simulink subsystem "VehicleSimulationRef"  (R2024b)
settings: Solver=VariableStepAuto  StartTime=0.0  StopTime=10.0  RelTol=1e-3
undefined symbols (not defined in the file): damp, flightTrajectory, Ka_accel, Kd_rate, Ki_angle, Kp_angle, omega, resetFlag, SimIn, SimPar, trajLen
libraries: starslibAxisTransformations x6, simulink_extras x5, dspstat3 x3, vrlib x3, aerolibanimutils x2, dspnetwork x1, aerolibfltsims x1, simulink x1
(part 1 of 2)
settings Model: Creator=tbritton  LastModifiedBy=edison
settings SolverCC: AlgebraicLoopSolver=TrustRegion
settings OptimizationCC: ReuseModelBlockBuffer=off
settings DebuggingCC: UnconnectedInputMsg=warning  UnconnectedOutputMsg=warning  UnconnectedLineMsg=warning
settings ModelReferenceCC: EnableRefExpFcnMdlSchedulingChecks=on
settings RTWCC: GPUComputeCapability=3.5  DLArmComputeVersion=19.05

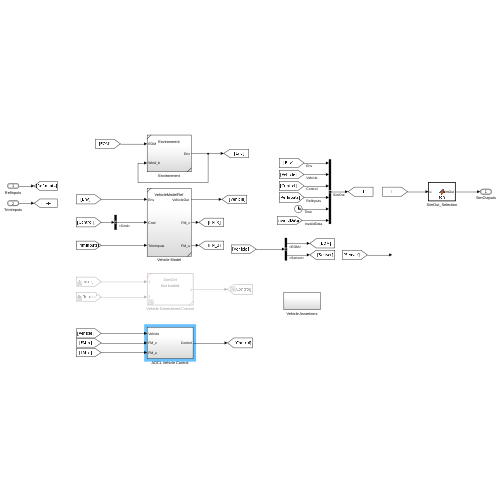
[thumbnail: Simulink's stored preview of the top-level diagram]
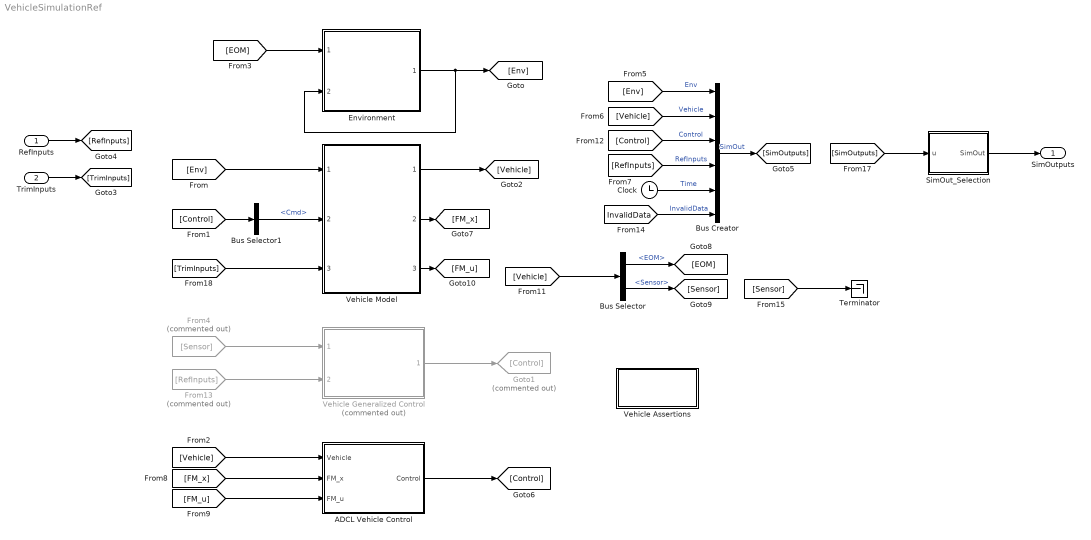
== system VehicleSimulationRef ==
  RefInputs : Inport  OutDataTypeStr=Bus: BUS_REF_INPUT
  TrimInputs : Inport  Port=2  OutDataTypeStr=Bus: BUS_TRIM_INPUT
  ADCL Vehicle Control : Subsystem
  Bus Creator : BusCreator  Inputs=6  OutDataTypeStr=Bus: BUS_SIM_OUT  NonVirtualBus=on
  Bus Selector : BusSelector  OutputSignals=EOM,Sensor
  Bus Selector1 : BusSelector  OutputSignals=Cmd
  Clock : Clock
  Environment : Subsystem  ReferencedSubsystem=Environment
  From13 : From  Commented=on  GotoTag=RefInputs
  From4 : From  Commented=on  GotoTag=Sensor
  Goto1 : Goto  Commented=on  GotoTag=Control
  SimOut_Selection : MATLAB Function  TreatAsAtomicUnit=on
  Terminator : Terminator
  Vehicle Assertions : Subsystem
  Vehicle Generalized Control : Subsystem  Commented=on  ReferencedSubsystem=GenCtrl
  Vehicle Model : Subsystem  ReferencedSubsystem=VehicleModelRef
  SimOutputs : Outport  OutDataTypeStr=Bus: BUS_USER_SIM_OUT
  wires:
  From4/1 -> Vehicle Generalized Control/1
  [Env] -> Bus Creator/1  "Env"
  [RefInputs] -> Bus Creator/4  "RefInputs"
  Environment/1 -> [Env], Environment/2
  Vehicle Generalized Control/1 -> Goto1/1
  [Vehicle] -> Bus Creator/2  "Vehicle"
  [Control] -> Bus Creator/3  "Control"
  Bus Selector/1 -> [EOM]  "<EOM>"
  [Vehicle] -> Bus Selector/1
  [EOM] -> Environment/1
  Bus Selector/2 -> [Sensor]  "<Sensor>"
  [Control] -> Bus Selector1/1
  From13/1 -> Vehicle Generalized Control/2
  Clock/1 -> Bus Creator/5  "Time"
  TrimInputs/1 -> [TrimInputs]
  RefInputs/1 -> [RefInputs]
  Bus Creator/1 -> [SimOutputs]  "SimOut"
  [InvalidData] -> Bus Creator/6  "InvalidData"
  [Env] -> Vehicle Model/1
  [TrimInputs] -> Vehicle Model/3
  Vehicle Model/1 -> [Vehicle]
  [SimOutputs] -> SimOut_Selection/1(u)
  SimOut_Selection/1(SimOut) -> SimOutputs/1
  [Vehicle] -> ADCL Vehicle Control/1(Vehicle)
  ADCL Vehicle Control/1(Control) -> [Control]
  [FM_x] -> ADCL Vehicle Control/2(FM_x)
  Vehicle Model/3 -> [FM_u]
  Vehicle Model/2 -> [FM_x]
  [FM_u] -> ADCL Vehicle Control/3(FM_u)
  [Sensor] -> Terminator/1
  Bus Selector1/1 -> Vehicle Model/2  "<Cmd>"

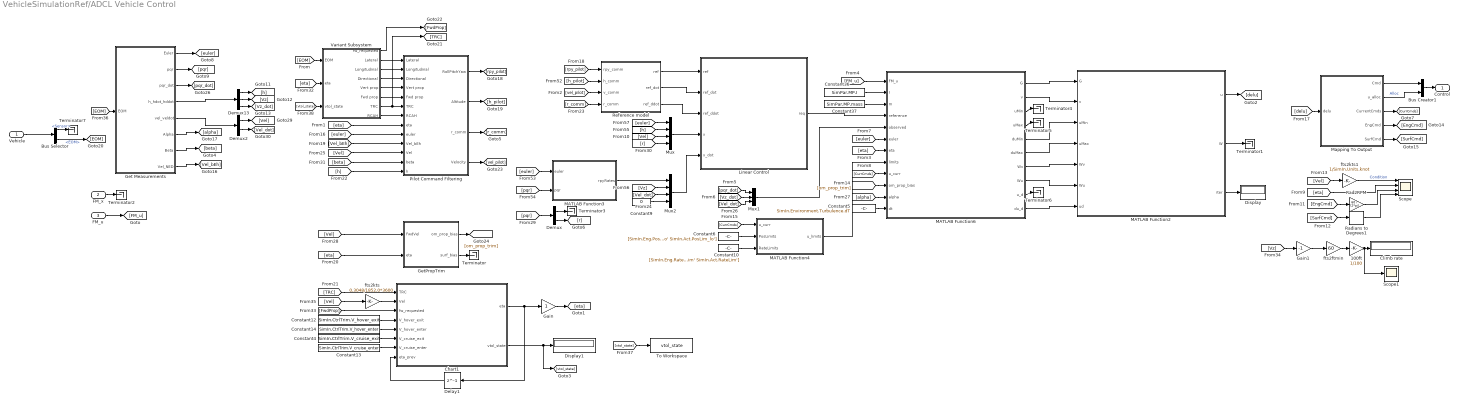
== system VehicleSimulationRef/ADCL Vehicle Control ==
  Vehicle : Inport
  FM_x : Inport  Port=2
  FM_u : Inport  Port=3
  100ft : Gain  Gain=1/100
  Bus Creator1 : BusCreator  Inputs=2
  Bus Selector : BusSelector  OutputSignals=Sensor,EOM
  Chart1 : Stateflow chart  TreatAsAtomicUnit=on
      settings: PortSchema="{\"entries\":[{\"content\":{\"sides\":[{\"content\":{\"connectorIds\":[\"In8\",\"In3\",\"In1\",\"In4\",\"In5\",\"In6\",\"In7\",\"In2\"]},\"type\":\"ConnectorPlacement.EquallySpacedRectSide\",\"uuid\":\"4afc29e3-93a7-44dd-bca0-17fa13a866cd\"},{\"content\":{\"connectorIds\":[\"Out1\",\"Out2\"],\"side\":\"RIGHT\"},\"type\":\"ConnectorPlacement.EquallySpacedRectSide\",\"uuid\":\"32f80fb4-c626-4840-bdaf-a1806a0598eb\"},{\"content\":{\"side\":\"TOP\"},\"type\":\"ConnectorPlacement.EquallySpacedRectSide\",\"uuid\":\"4ca4e56e-6e18-44cf-80c6-f56236f2c6df\"}]},\"type\":\"ConnectorPlacement.EquallySpacedConnector\",\"uuid\":\"a5138527-01bf-491a-89e0-3407f8ac8af7\"}],\"packageUris\":[\"http://schema.mathworks.com/mf0/Connector/R2020b\"],\"version\":\"1.0\"}"
  Climb rate : Display
  Constant10 : Constant  Value=[SimIn.Eng.RateLim' SimIn.Act.RateLim']
  Constant12 : Constant  Value=SimIn.CtrlTrim.V_hover_exit
  Constant13 : Constant  Value=SimIn.CtrlTrim.V_cruise_enter
  Constant14 : Constant  Value=SimIn.CtrlTrim.V_hover_enter
  Constant36 : Constant  Value=SimPar.MP.I
  Constant37 : Constant  Value=SimPar.MP.mass
  Constant4 : Constant  Value=SimIn.CtrlTrim.V_cruise_exit
  Constant5 : Constant  Value=SimIn.Environment.Turbulence.dT
  Constant6 : Constant  Value=[SimIn.Eng.PosLim_hi' SimIn.Act.PosLim_hi'; SimIn.Eng.PosLim_lo' SimIn.Act.PosLim_lo']
  Constant9 : Constant  Value=0
  Delay1 : Delay  DelayLength=1
  Demux : Demux  Outputs=[2 1]
  Demux13 : Demux  Outputs=3
  Demux2 : Demux  Outputs=2
  Display : Display
  Display1 : Display
  Gain : Gain
  Gain1 : Gain  Gain=-1
  Get Measurements : Subsystem
  GetPropTrim : Subsystem
  Linear Control : Subsystem  mask{Krp_angle=5, Krp_angle_i=3, Krp_rate=5, Krp_accel=1, Ky_angle=0.75, Ky_rate=2.5, Ky_accel=0.75, Kr_rate=2, Kh_angle=0.8, Kh_rate=2, Kh_accel=1}
      mask prompts: Krp_angle "Roll and Pitch angle gain"; Krp_angle_i "Roll and Pitch angle gain integral"; Krp_rate "Roll and Pitch rate gain"; Krp_accel "Roll and Pitch accel. gain"; Ky_angle "Yaw angle gain"; Ky_rate "Yaw rate gain"; Ky_accel "Yaw accel. gain"; Kr_rate "Turn coord. rate gain"; Kh_angle "Altitude angle gain"; Kh_rate "Altitude rate gain"; Kh_accel "Altitude accel. gain"
      mask DialogControl DescTextVar Prompt: Linear controller gains
      mask DialogControl Container3 Prompt: Roll and Pitch
      mask DialogControl Container4 Prompt: Yaw
      mask DialogControl Container5 Prompt: Altitude and Forward vel.
  MATLAB Function2 : MATLAB Function  TreatAsAtomicUnit=on
  MATLAB Function3 : MATLAB Function  TreatAsAtomicUnit=on
  MATLAB Function4 : MATLAB Function  TreatAsAtomicUnit=on
  MATLAB Function6 : MATLAB Function  TreatAsAtomicUnit=on
  Mapping To Output : Subsystem
  Mux : Mux
  Mux1 : Mux  Inputs=3
  Mux2 : Mux
  Pilot Command Filtering : Subsystem  mask{Vel_TRC=SimIn.CtrlTrim.V_TRC}
      mask prompts: Vel_TRC "TRC Velocity Threshold"
      mask DialogControl DescTextVar Prompt: Pilot command filtering depending on the flight condition
  Rad2RPM : Gain  Gain=60 / (2*pi)
  Radians to Degrees1 : simulink_extras/Transformations/Radians to Degrees
  Reference model : Subsystem  mask{r_omega=1.4, r_damp=0.8, p_omega=2.4, p_damp=0.8, y_omega=0.67, y_damp=0.8, h_omega=0.67, h_damp=0.8}
      mask prompts: r_omega "Roll natural freq."; r_damp "Roll damping ratio"; p_omega "Pitch natural freq."; p_damp "Pitch damping ratio"; y_omega "Yaw natural freq."; y_damp "Yaw damping ratio"; h_omega "Altitude natural freq."; h_damp "Altitude damping ratio"
      mask DialogControl DescTextVar Prompt: Second order reference models for the roll, pitch, yaw and altitude channles
      mask DialogControl Container3 Prompt: Roll parameters
      mask DialogControl Container4 Prompt: Pitch parameters
      mask DialogControl Container5 Prompt: Yaw parameters
      mask DialogControl Container6 Prompt: Altitude parameters
  Scope : Scope  NumInputPorts=4
  Scope1 : Scope
  Terminator{,1..7} (8 alike) : Terminator
  To Workspace : ToWorkspace  VariableName=vtol_state  SaveFormat=Timeseries  SampleTime=-1
  Variant Subsystem : Subsystem  Variant=on
  fts2ftmin : Gain  Gain=60
  fts2kts : Gain  Gain=0.3048/1852.0*3600
  fts2kts1 : Gain  Gain=1/SimIn.Units.knot
  Control : Outport
  wires:
  Bus Selector/1 -> Terminator7/1  "<Sensor>"
  Get Measurements/2(pqr) -> [pqr]
  Get Measurements/5(vel_veldot) -> Demux2/1
  Get Measurements/4(h_hdot_hddot) -> Demux13/1
  Get Measurements/8(Vel_NED) -> [Vel_bEh]
  Get Measurements/7(Beta) -> [beta]
  Get Measurements/6(Alpha) -> [alpha]
  Get Measurements/3(pqr_dot) -> [pqr_dot]
  Get Measurements/1(Euler) -> [euler]
  [Vel_dot] -> Mux1/3
  [EOM] -> Get Measurements/1(EOM)
  Bus Selector/2 -> [EOM]  "<EOM>"
  Vehicle/1 -> Bus Selector/1
  [Vel] -> fts2kts/1
  [TRC] -> Chart1/8(TRC)
  [eta] -> GetPropTrim/2(eta)
  [vtol_state] -> Variant Subsystem/3(vtol_state)
  [vtol_state] -> To Workspace/1
  [rpy_pilot] -> Reference model/1(rpy_comm)
  Gain/1 -> [eta]
  Variant Subsystem/1(fw_requested) -> [FwdProp]
  Chart1/2(vtol_state) -> Display1/1, [vtol_state]
  MATLAB Function6/8(Wu) -> MATLAB Function2/6(Wu)
  Variant Subsystem/8(RCAH) -> Pilot Command Filtering/7(RCAH)
  Variant Subsystem/6(Fwd prop) -> Pilot Command Filtering/5(Fwd prop)
  Variant Subsystem/5(Vert prop) -> Pilot Command Filtering/4(Vert prop)
  Variant Subsystem/4(Directional) -> Pilot Command Filtering/3(Directional)
  Variant Subsystem/3(Longitudinal) -> Pilot Command Filtering/2(Longitudinal)
  Variant Subsystem/2(Lateral) -> Pilot Command Filtering/1(Lateral)
  [FwdProp] -> Chart1/1(fw_requested)
  Rad2RPM/1 -> Scope/3
  Chart1/1(eta) -> Gain/1, Delay1/1
  Delay1/1 -> Chart1/2(eta_prev)
  Constant12/1 -> Chart1/4(V_hover_exit)
  Constant14/1 -> Chart1/5(V_hover_enter)
  Constant13/1 -> Chart1/7(V_cruise_enter)
  Constant4/1 -> Chart1/6(V_cruise_exit)
  [eta] -> Variant Subsystem/2(eta)
  GetPropTrim/1(om_prop_bias) -> [om_prop_trim]
  [h] -> Pilot Command Filtering/13(h)
  Variant Subsystem/7(TRC) -> Pilot Command Filtering/6(TRC), [TRC]
  GetPropTrim/2(surf_bias) -> Terminator/1
  [Vel] -> GetPropTrim/1(FwdVel)
  [EOM] -> Variant Subsystem/1(EOM)
  Reference model/2(ref_dot) -> Linear Control/2(ref_dot)
  Linear Control/1(req) -> MATLAB Function6/4(reference)
  fts2kts/1 -> Chart1/3(Vel)
  fts2kts1/1 -> Scope/1  "Condition"
  [beta] -> Pilot Command Filtering/12(beta)
  Pilot Command Filtering/3(r_comm) -> [r_comm]
  [Vel] -> Pilot Command Filtering/11(Vel)
  [Vel_bEh] -> Pilot Command Filtering/10(Vel_bEh)
  MATLAB Function6/3(uMin) -> Terminator4/1
  MATLAB Function6/4(uMax) -> Terminator5/1
  MATLAB Function6/9(u_d) -> Terminator6/1
  Pilot Command Filtering/1(RollPitchYaw) -> [rpy_pilot]
  Pilot Command Filtering/2(Altitude) -> [h_pilot]
  Pilot Command Filtering/4(Velocity) -> [vel_pilot]
  [euler] -> Pilot Command Filtering/9(euler)
  [eta] -> Pilot Command Filtering/8(eta)
  [h] -> Mux/2
  Mux/1 -> Linear Control/4(x)
  [h_pilot] -> Reference model/2(h_comm)
  Reference model/3(ref_ddot) -> Linear Control/3(ref_ddot)
  [euler] -> MATLAB Function3/1(euler)
  Mux2/1 -> Linear Control/5(x_dot)
  Reference model/1(ref) -> Linear Control/1(ref)
  [pqr] -> MATLAB Function3/2(pqr)
  [euler] -> Mux/1
  [Vz] -> Mux2/2
  MATLAB Function3/1(rpyRates) -> Mux2/1
  Bus Creator1/1 -> Control/1
  FM_x/1 -> Terminator2/1
  FM_u/1 -> [FM_u]
  [FM_u] -> MATLAB Function6/1(FM_u)
  Constant36/1 -> MATLAB Function6/2(I)
  Constant37/1 -> MATLAB Function6/3(m)
  [eta] -> MATLAB Function6/7(eta)
  [euler] -> MATLAB Function6/6(euler)
  MATLAB Function6/2(v) -> MATLAB Function2/2(v)
  [eta] -> Scope/2
  [SurfCmd] -> Radians to Degrees1/1
  [EngCmd] -> Rad2RPM/1
  Radians to Degrees1/1 -> Scope/4
  Demux13/1 -> [h]
  Demux13/2 -> [Vz]
  Demux13/3 -> [Vz_dot]
  [om_prop_trim] -> MATLAB Function6/10(om_prop_bias)
  Mapping To Output/1(Cmd) -> Bus Creator1/1
  Mapping To Output/2(u_alloc) -> Bus Creator1/2  "Alloc"
  Mapping To Output/3(CurrentCmds) -> [CurrCmds]
  [CurrCmds] -> MATLAB Function6/9(u_curr)
  Mapping To Output/5(SurfCmd) -> [SurfCmd]
  Mapping To Output/4(EngCmd) -> [EngCmd]
  Demux2/2 -> [Vel_dot]
  Demux2/1 -> [Vel]
  [Vel] -> Mux/3
  [Vel_dot] -> Mux2/3
  [alpha] -> MATLAB Function6/11(alpha)
  MATLAB Function6/1(G) -> MATLAB Function2/1(G)
  MATLAB Function6/7(Wv) -> MATLAB Function2/5(Wv)
  MATLAB Function6/5(duMin) -> MATLAB Function2/3(uMin)
  MATLAB Function6/6(duMax) -> MATLAB Function2/4(uMax)
  [Vz_dot] -> Mux1/2
  [pqr_dot] -> Mux1/1
  Constant5/1 -> MATLAB Function6/12(dt)
  [vel_pilot] -> Reference model/3(v_comm)
  Constant6/1 -> MATLAB Function4/2(PosLimits)
  MATLAB Function4/1(u_limits) -> MATLAB Function6/8(limits)
  MATLAB Function6/10(du_d) -> MATLAB Function2/7(ud)
  [Vel] -> fts2kts1/1
  MATLAB Function2/3(iter) -> Display/1
  MATLAB Function2/2(W) -> Terminator1/1
  [delu] -> Mapping To Output/1(delu)
  [CurrCmds] -> MATLAB Function4/1(u_curr)
  Mux1/1 -> MATLAB Function6/5(observed)
  MATLAB Function2/1(u) -> [delu]
  Constant10/1 -> MATLAB Function4/3(RateLimits)
  [r_comm] -> Reference model/4(r_comm)
  [pqr] -> Demux/1
  Demux/2 -> [r]
  Demux/1 -> Terminator3/1
  [r] -> Mux/4
  Constant9/1 -> Mux2/4
  Gain1/1 -> fts2ftmin/1
  100ft/1 -> Climb rate/1, Scope1/1
  fts2ftmin/1 -> 100ft/1
  [Vz] -> Gain1/1

== system VehicleSimulationRef/Vehicle Assertions ==
  Clock1 : Clock
  Compare To Constant : simulink/Logic and Bit Operations/Compare To Constant  relop=>=  const=0.2  OutDataTypeStr=boolean  ZeroCross=off
  Demux : Demux  Outputs=2
  KillifNotValidPropSpd : Assertion  AssertionFailFcn=warndlg('Model invalid prop speeds','Warning!')
  KillifNotValidSpd : Assertion  AssertionFailFcn=warndlg('Model invalid speed','Warning!')
  Logical Operator : Logic  Operator=NAND  AllPortsSameDT=off  OutDataTypeStr=boolean
  Logical Operator1 : Logic  Operator=NAND  AllPortsSameDT=off  OutDataTypeStr=boolean
  Logical Operator2 : Logic  Operator=OR  AllPortsSameDT=off  OutDataTypeStr=boolean
  tag scope: InvalidData=global
  wires:
  [InvalidPropSpd] -> Logical Operator2/2
  [InvalidSpd] -> Logical Operator2/1
  Logical Operator2/1 -> [InvalidData]
  Logical Operator/1 -> KillifNotValidSpd/1
  [InvalidPropSpd] -> Logical Operator1/1
  Logical Operator1/1 -> KillifNotValidPropSpd/1
  [Time] -> Logical Operator1/2
  [Time] -> Logical Operator/2
  Compare To Constant/1 -> [Time]
  Demux/2 -> [InvalidPropSpd]
  Demux/1 -> [InvalidSpd]
  [Validity] -> Demux/1
  [InvalidSpd] -> Logical Operator/1
  Clock1/1 -> Compare To Constant/1

== system VehicleSimulationRef/ADCL Vehicle Control/Get Measurements ==
  EOM : Inport
  Bus Selector3 : BusSelector  OutputSignals=WorldRelativeData.Euler.phi,WorldRelativeData.Euler.theta,WorldRelativeData.Euler.psi,InertialData.Omeg_BIb,InertialData.OmegDtI_BIb,InertialData.Pos_bii,InertialData.Vel_bIi,InertialData.Accel_bIi,AirRelativeData.Vtot,AirRelativeData.Vtotdot,AirRelativeData.alpha,AirRelativeData.beta,WorldRelativeData.Vel_bEh
  Demux11 : Demux  Outputs=[2 1]
  Demux7 : Demux  Outputs=[2 1]
  Demux8 : Demux  Outputs=[2 1]
  Mux : Mux  Inputs=3
  Mux1 : Mux  Inputs=2
  Mux3 : Mux  Inputs=3
  Terminator1 : Terminator
  Terminator10 : Terminator
  Terminator6 : Terminator
  To Workspace : ToWorkspace  VariableName=headingNED_W  SaveFormat=Timeseries  SampleTime=-1
      settings: MaxDataPoints=1
  To Workspace1 : ToWorkspace  VariableName=NEDpos_W  SaveFormat=Timeseries  SampleTime=-1
      settings: MaxDataPoints=1  Save2DSignal=2-D array (concatenate along first dimension)
  Euler : Outport
  pqr : Outport  Port=2
  pqr_dot : Outport  Port=3
  h_hdot_hddot : Outport  Port=4
  vel_veldot : Outport  Port=5
  Alpha : Outport  Port=6
  Beta : Outport  Port=7
  Vel_NED : Outport  Port=8
  wires:
  Bus Selector3/13 -> Vel_NED/1  "<Vel_bEh>"
  Demux8/1 -> Terminator1/1
  Bus Selector3/7 -> Demux8/1  "<Vel_bIi>"
  Bus Selector3/6 -> Demux7/1, To Workspace1/1  "<Pos_bii>"
  EOM/1 -> Bus Selector3/1
  Demux7/1 -> Terminator6/1
  Bus Selector3/8 -> Demux11/1  "<Accel_bIi>"
  Bus Selector3/1 -> Mux3/1  "<phi>"
  Demux11/1 -> Terminator10/1
  Demux11/2 -> Mux/3
  Demux7/2 -> Mux/1
  Bus Selector3/2 -> Mux3/2  "<theta>"
  Bus Selector3/3 -> Mux3/3, To Workspace/1  "<psi>"
  Mux3/1 -> Euler/1
  Bus Selector3/4 -> pqr/1  "<Omeg_BIb>"
  Bus Selector3/5 -> pqr_dot/1  "<OmegDtI_BIb>"
  Mux/1 -> h_hdot_hddot/1
  Demux8/2 -> Mux/2
  Bus Selector3/11 -> Alpha/1  "<alpha>"
  Bus Selector3/10 -> Mux1/2  "<Vtotdot>"
  Bus Selector3/9 -> Mux1/1  "<Vtot>"
  Mux1/1 -> vel_veldot/1
  Bus Selector3/12 -> Beta/1  "<beta>"

== system VehicleSimulationRef/ADCL Vehicle Control/GetPropTrim ==
  FwdVel : Inport
  eta : Inport  Port=2
  Constant : Constant  Value=0
  Constant8 : Constant
  Demux12 : Demux  Outputs=[10 1 1 4 SimIn.numEngines]
  Matrix Interpolation1 : simulink_extras/Additional Lookup Tables/Matrix Interpolation  InterpMethod=Linear  ExtrapMethod=Clip  InterpolateDimension=2  TableData=SimIn.Control.trim.XU0_interp  SimulateUsing=Code generation
  Prelookup : PreLookup  BreakpointsData=SimIn.Control.trim.UH
  Prelookup1 : PreLookup  BreakpointsData=SimIn.Control.trim.WH
  Product : Product
  Product1 : Product
  Saturation : Saturate  UpperLimit=max(SimIn.Control.trim.UH)  LowerLimit=0
  Saturation3 : Saturate  UpperLimit=8.33  LowerLimit=-8.33
  Selector : Selector  InputPortWidth=SimIn.numEngines  IndexOptions=Index vector (dialog)  Indices=SimIn.numEngines  OutputSizes=1
  Selector1 : Selector  InputPortWidth=SimIn.numEngines  IndexOptions=Index vector (dialog)  Indices=1:SimIn.numEngines-1  OutputSizes=1
  Sum : Sum  Inputs=|+-
  Terminator : Terminator
  Terminator1 : Terminator
  Terminator2 : Terminator
  Transpose1 : Math  Operator=transpose
  VTOLScale : Gain  Gain=1/sqrt(SimPar.Scale)
  Vector Concatenate : Concatenate
  om_prop_bias : Outport
  surf_bias : Outport  Port=2
  wires:
  Demux12/2 -> Terminator2/1
  eta/1 -> [eta]
  Product1/1 -> Vector Concatenate/1
  Constant8/1 -> Sum/1
  Selector1/1 -> Product1/1
  Selector/1 -> Product/1
  Product/1 -> Vector Concatenate/2
  [eta] -> Sum/2
  [eta] -> Product1/2
  VTOLScale/1 -> Selector1/1, Selector/1
  Vector Concatenate/1 -> om_prop_bias/1
  Sum/1 -> Product/2
  Matrix Interpolation1/1 -> Transpose1/1
  Demux12/3 -> Terminator1/1
  Demux12/5 -> VTOLScale/1
  Demux12/4 -> surf_bias/1
  Constant/1 -> Saturation3/1
  Prelookup/1 -> Matrix Interpolation1/1
  Prelookup1/1 -> Matrix Interpolation1/3
  Demux12/1 -> Terminator/1
  Prelookup/2 -> Matrix Interpolation1/2
  Prelookup1/2 -> Matrix Interpolation1/4
  Transpose1/1 -> Demux12/1
  Saturation/1 -> Prelookup/1
  Saturation3/1 -> Prelookup1/1
  FwdVel/1 -> Saturation/1

== system VehicleSimulationRef/ADCL Vehicle Control/Linear Control ==
  ref : Inport
  ref_dot : Inport  Port=2
  ref_ddot : Inport  Port=3
  x : Inport  Port=4
  x_dot : Inport  Port=5
  Gain : Gain  Gain=Kp_angle
  Gain1 : Gain  Gain=Ki_angle
  Gain2 : Gain  Gain=Kd_rate
  Gain3 : Gain  Gain=Ka_accel
  Integrator : Integrator  LimitOutput=on  UpperSaturationLimit=[0.7; 0.7; 0.7; inf; inf; 0.7]  LowerSaturationLimit=-[0.7; 0.7; 0.7; inf; inf; 0.7]
  Sum : Sum  Inputs=|+-
  Sum1 : Sum  Inputs=|+-
  Sum2 : Sum  Inputs=+++
  Sum3 : Sum  Inputs=|++
  req : Outport
  wires:
  Gain2/1 -> Sum2/2
  Sum2/1 -> req/1
  ref/1 -> Sum/1
  x/1 -> Sum/2
  Gain1/1 -> Integrator/1
  Sum/1 -> Gain/1, Gain1/1
  ref_dot/1 -> Sum1/1
  Sum1/1 -> Gain2/1
  x_dot/1 -> Sum1/2
  ref_ddot/1 -> Gain3/1
  Gain3/1 -> Sum2/3
  Gain/1 -> Sum3/1
  Integrator/1 -> Sum3/2
  Sum3/1 -> Sum2/1

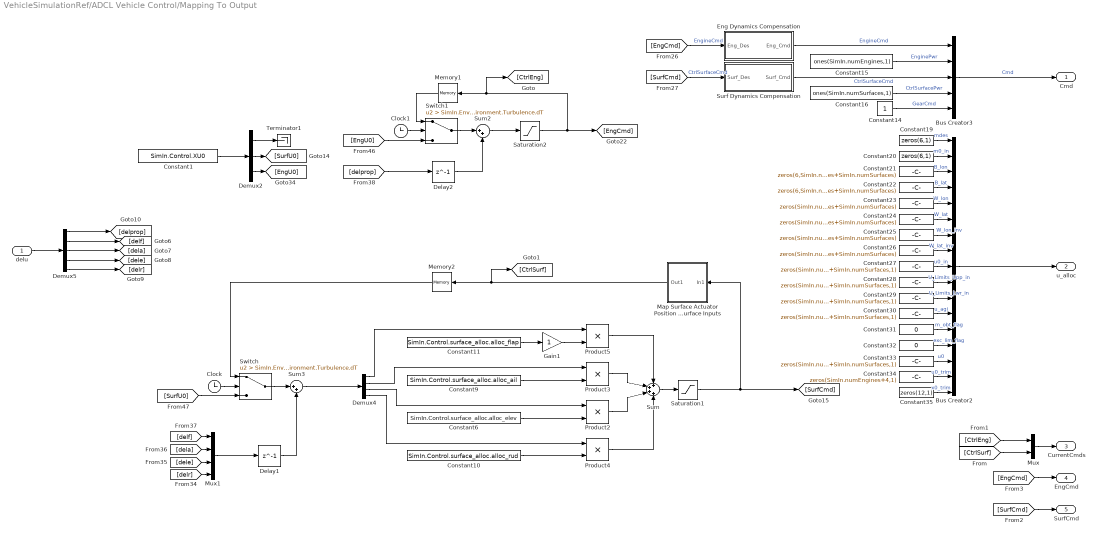
== system VehicleSimulationRef/ADCL Vehicle Control/Mapping To Output ==
  delu : Inport
  Bus Creator2 : BusCreator  Inputs=17  OutDataTypeStr=Bus: BUS_ALLOC
  Bus Creator3 : BusCreator  Inputs=5  OutDataTypeStr=Bus: BUS_CMD
  Clock : Clock
  Clock1 : Clock
  Constant1 : Constant  Value=SimIn.Control.XU0
  Constant10 : Constant  Value=SimIn.Control.surface_alloc.alloc_rud
  Constant11 : Constant  Value=SimIn.Control.surface_alloc.alloc_flap
  Constant14 : Constant
  Constant15 : Constant  Value=ones(SimIn.numEngines,1)
  Constant16 : Constant  Value=ones(SimIn.numSurfaces,1)
  Constant19 : Constant  Value=zeros(6,1)
  Constant20 : Constant  Value=zeros(6,1)
  Constant21 : Constant  Value=zeros(6,SimIn.numEngines+SimIn.numSurfaces)
  Constant22 : Constant  Value=zeros(6,SimIn.numEngines+SimIn.numSurfaces)
  Constant{23..26} (4 alike) : Constant  Value=zeros(SimIn.numEngines+SimIn.numSurfaces)
  Constant{27..30,33} (5 alike) : Constant  Value=zeros(SimIn.numEngines+SimIn.numSurfaces,1)
  Constant31 : Constant  Value=0
  Constant32 : Constant  Value=0
  Constant34 : Constant  Value=zeros(SimIn.numEngines+4,1)
  Constant35 : Constant  Value=zeros(12,1)
  Constant6 : Constant  Value=SimIn.Control.surface_alloc.alloc_elev
  Constant9 : Constant  Value=SimIn.Control.surface_alloc.alloc_ail
  Delay1 : Delay  DelayLength=1
  Delay2 : Delay  DelayLength=1
  Demux2 : Demux  Outputs=[-1 4 SimIn.numEngines]
  Demux4 : Demux
  Demux5 : Demux  Outputs=[SimIn.numEngines 1 1 1 1]
  Eng Dynamics Compensation : Subsystem  Variant=on
  Gain1 : Gain
  Map Surface Actuator Position To Surface Inputs : Subsystem
  Memory1 : Memory
  Memory2 : Memory
  Mux : Mux  Inputs=2
  Mux1 : Mux
  Product{2..5} (4 alike) : Product
  Saturation1 : Saturate  UpperLimit=SimPar.Actuator.MaxPos  LowerLimit=SimPar.Actuator.MinPos
  Saturation2 : Saturate  UpperLimit=SimPar.Engine.MaxPos  LowerLimit=SimPar.Engine.MinPos
  Sum : Sum  Inputs=++++
  Sum2 : Sum  Inputs=|++
  Sum3 : Sum  Inputs=|++
  Surf Dynamics Compensation : Subsystem  Variant=on
  Switch : Switch  Criteria=u2 > Threshold  Threshold=SimIn.Environment.Turbulence.dT  SaturateOnIntegerOverflow=off  InputSameDT=off
  Switch1 : Switch  Criteria=u2 > Threshold  Threshold=SimIn.Environment.Turbulence.dT  SaturateOnIntegerOverflow=off  InputSameDT=off
  Terminator1 : Terminator
  Cmd : Outport
  u_alloc : Outport  Port=2
  CurrentCmds : Outport  Port=3
  EngCmd : Outport  Port=4
  SurfCmd : Outport  Port=5
  wires:
  Delay1/1 -> Sum3/2
  [CtrlSurf] -> Mux/2
  [CtrlEng] -> Mux/1
  Map Surface Actuator Position To Surface Inputs/1(Out1) -> Memory2/1, [CtrlSurf]
  Delay2/1 -> Sum2/2
  Memory1/1 -> Switch1/1
  Memory2/1 -> Switch/1
  Mux1/1 -> Delay1/1
  [delprop] -> Delay2/1
  Saturation2/1 -> [EngCmd], Memory1/1, [CtrlEng]
  Eng Dynamics Compensation/1(Eng_Cmd) -> Bus Creator3/1  "EngineCmd"
  Surf Dynamics Compensation/1(Surf_Cmd) -> Bus Creator3/3  "CtrlSurfaceCmd"
  Constant6/1 -> Product2/2
  Switch/1 -> Sum3/1
  Bus Creator3/1 -> Cmd/1  "Cmd"
  Demux4/2 -> Product3/1
  Constant31/1 -> Bus Creator2/13  "m_obt_flag"
  [SurfCmd] -> Surf Dynamics Compensation/1(Surf_Des)  "CtrlSurfaceCmd"
  [SurfU0] -> Switch/3
  Constant26/1 -> Bus Creator2/8  "W_lat_inv"
  Demux4/4 -> Product4/1
  Constant9/1 -> Product3/2
  [EngCmd] -> Eng Dynamics Compensation/1(Eng_Des)  "EngineCmd"
  Product5/1 -> Sum/1
  [delf] -> Mux1/1
  Constant24/1 -> Bus Creator2/6  "W_lat"
  [dela] -> Mux1/2
  Product2/1 -> Sum/3
  Demux2/1 -> Terminator1/1
  [delr] -> Mux1/4
  Sum/1 -> Saturation1/1
  Constant19/1 -> Bus Creator2/1  "mdes"
  Constant22/1 -> Bus Creator2/4  "B_lat"
  Constant33/1 -> Bus Creator2/15  "u0"
  Switch1/1 -> Sum2/1
  Product4/1 -> Sum/4
  Constant20/1 -> Bus Creator2/2  "m0_in"
  Constant28/1 -> Bus Creator2/10  "U_Limits_Upp_in"
  Gain1/1 -> Product5/2
  Clock1/1 -> Switch1/2
  Demux2/2 -> [SurfU0]
  Demux4/3 -> Product2/1
  Clock/1 -> Switch/2
  Constant16/1 -> Bus Creator3/4  "CtrlSurfacePwr"
  Demux2/3 -> [EngU0]
  Constant27/1 -> Bus Creator2/9  "u0_in"
  Constant11/1 -> Gain1/1
  Saturation1/1 -> [SurfCmd], Map Surface Actuator Position To Surface Inputs/1(In1)
  [EngU0] -> Switch1/3
  Constant29/1 -> Bus Creator2/11  "U_Limits_Lwr_in"
  Constant1/1 -> Demux2/1
  [dele] -> Mux1/3
  Product3/1 -> Sum/2
  Constant32/1 -> Bus Creator2/14  "exc_lim_flag"
  Bus Creator2/1 -> u_alloc/1
  Constant15/1 -> Bus Creator3/2  "EnginePwr"
  Constant30/1 -> Bus Creator2/12  "u_agi"
  Sum3/1 -> Demux4/1
  Constant25/1 -> Bus Creator2/7  "W_lon_inv"
  Demux4/1 -> Product5/1
  Constant35/1 -> Bus Creator2/17  "x0_trim"
  Constant14/1 -> Bus Creator3/5  "GearCmd"
  Constant23/1 -> Bus Creator2/5  "W_lon"
  Constant21/1 -> Bus Creator2/3  "B_lon"
  Constant10/1 -> Product4/2
  Constant34/1 -> Bus Creator2/16  "u0_trim"
  Sum2/1 -> Saturation2/1
  Mux/1 -> CurrentCmds/1
  [SurfCmd] -> SurfCmd/1
  [EngCmd] -> EngCmd/1
  Demux5/2 -> [delf]
  delu/1 -> Demux5/1
  Demux5/1 -> [delprop]
  Demux5/3 -> [dela]
  Demux5/4 -> [dele]
  Demux5/5 -> [delr]

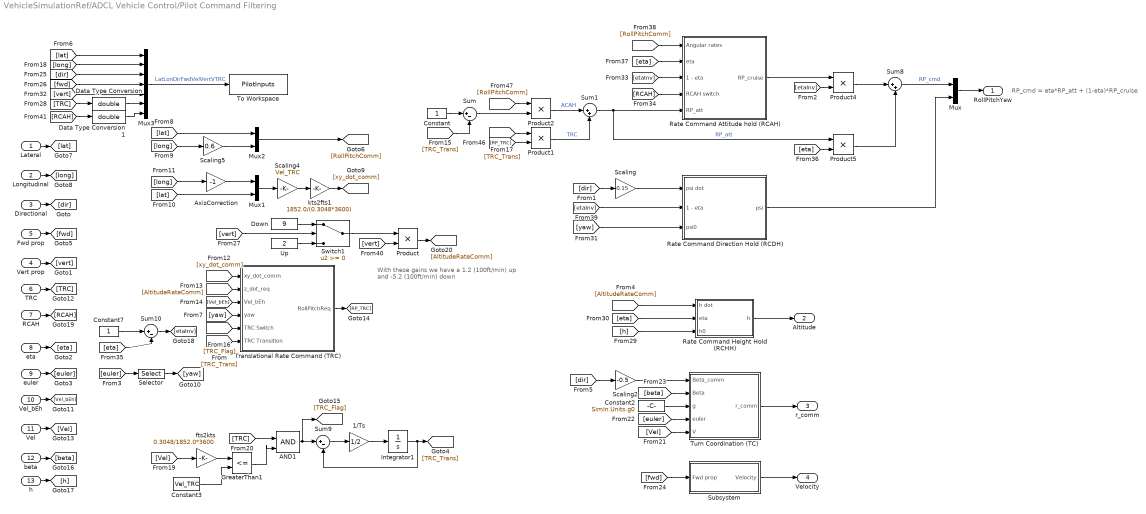
== system VehicleSimulationRef/ADCL Vehicle Control/Pilot Command Filtering ==
  note: RP_cmd = eta*RP_att + (1-eta)*RP_cruise
  note: With these gains we have a 1.2 (100ft/min) up
      | and -5.2 (100ft/min) down
  Lateral : Inport
  Longitudinal : Inport  Port=2
  Directional : Inport  Port=3
  Vert prop : Inport  Port=4
  Fwd prop : Inport  Port=5
  TRC : Inport  Port=6
  RCAH : Inport  Port=7
  eta : Inport  Port=8
  euler : Inport  Port=9
  Vel_bEh : Inport  Port=10
  Vel : Inport  Port=11
  beta : Inport  Port=12
  h : Inport  Port=13
  1/Ts : Gain  Gain=1/2
  AND1 : Logic  IconShape=distinctive  AllPortsSameDT=off  OutDataTypeStr=boolean
  AxisCorrection : Gain  Gain=-1
  Constant : Constant
  Constant2 : Constant  Value=SimIn.Units.g0
  Constant3 : Constant  Value=Vel_TRC
  Constant7 : Constant
  Data Type Conversion : DataTypeConversion  OutDataTypeStr=double  SaturateOnIntegerOverflow=off  RndMeth=Floor
  Data Type Conversion1 : DataTypeConversion  OutDataTypeStr=double  SaturateOnIntegerOverflow=off  RndMeth=Floor
  Down : Constant  Value=9
  GreaterThan1 : RelationalOperator  Operator=<=  OutDataTypeStr=boolean  RndMeth=Simplest  InputSameDT=off
  Integrator1 : Integrator
  Mux : Mux  Inputs=2
  Mux1 : Mux  Inputs=2
  Mux2 : Mux  Inputs=2
  Mux3 : Mux  Inputs=7
  Product{,1..2,4..5} (5 alike) : Product
  Rate Command Attitude hold (RCAH) : Subsystem
  Rate Command Direction Hold (RCDH) : Subsystem
  Rate Command Height Hold (RCHH) : Subsystem
  Scaling : Gain  Gain=0.15
  Scaling2 : Gain  Gain=-0.5
  Scaling4 : Gain  Gain=Vel_TRC
  Scaling5 : Gain  Gain=0.6
  Selector : Selector  InputPortWidth=3  IndexOptions=Index vector (dialog)  Indices=3  OutputSizes=1
  Subsystem : Subsystem
  Sum : Sum  Inputs=|+-
  Sum1 : Sum  Inputs=|++
  Sum10 : Sum  Inputs=|+-
  Sum8 : Sum  Inputs=|++
  Sum9 : Sum  Inputs=|+-
  Switch1 : Switch  SaturateOnIntegerOverflow=off  InputSameDT=off
  To Workspace : ToWorkspace  VariableName=PilotInputs  SaveFormat=Structure With Time  SampleTime=-1
  Translational Rate Command (TRC) : Subsystem
  Turn Coordination (TC) : Subsystem  mask{Kbeta=0.5}
      mask prompts: Kbeta "Controller gain"
      mask DialogControl DescTextVar Prompt: Sideslip control for turn coordination
  Up : Constant  Value=2
  fts2kts : Gain  Gain=0.3048/1852.0*3600
  kts2fts1 : Gain  Gain=1852.0/(0.3048*3600)
  RollPitchYaw : Outport
  Altitude : Outport  Port=2
  r_comm : Outport  Port=3
  Velocity : Outport  Port=4
  wires:
  [TRC_Trans] -> Product1/1
  [TRC_Trans] -> Sum/2
  [TRC_Trans] -> Translational Rate Command (TRC)/6(TRC Transition)
  [lat] -> Mux2/1
  Product1/1 -> Sum1/2  "TRC"
  Product2/1 -> Sum1/1  "ACAH"
  [RollPitchComm] -> Product2/1
  [RP_TRC] -> Product1/2
  Sum/1 -> Product2/2
  Constant/1 -> Sum/1
  Sum9/1 -> 1/Ts/1
  Integrator1/1 -> Sum9/2, [TRC_Trans]
  1/Ts/1 -> Integrator1/1
  Data Type Conversion1/1 -> Mux3/7
  [RCAH] -> Data Type Conversion1/1
  [vert] -> Product/2
  Switch1/1 -> Product/1
  Product/1 -> [AltitudeRateComm]
  Down/1 -> Switch1/1
  Up/1 -> Switch1/3
  [RCAH] -> Rate Command Attitude hold (RCAH)/4(RCAH switch)
  RCAH/1 -> [RCAH]
  Product4/1 -> Sum8/1
  Product5/1 -> Sum8/2
  Rate Command Attitude hold (RCAH)/1(RP_cruise) -> Product4/1
  [etaInv] -> Rate Command Attitude hold (RCAH)/3(1 - eta)
  [eta] -> Rate Command Attitude hold (RCAH)/2(eta)
  [RollPitchComm] -> Rate Command Attitude hold (RCAH)/1(Angular rates)
  [etaInv] -> Product4/2
  [etaInv] -> Rate Command Direction Hold (RCDH)/2(1 - eta)
  Sum10/1 -> [etaInv]
  [eta] -> Sum10/2
  Constant7/1 -> Sum10/1
  Sum8/1 -> Mux/1  "RP_cmd"
  Sum1/1 -> Rate Command Attitude hold (RCAH)/5(RP_att), Product5/1  "RP_att"
  [eta] -> Product5/2
  Mux2/1 -> [RollPitchComm]
  Scaling5/1 -> Mux2/2
  [vert] -> Switch1/2
  Vert prop/1 -> [vert]
  Scaling/1 -> Rate Command Direction Hold (RCDH)/1(psi dot)
  Selector/1 -> [yaw]
  [euler] -> Selector/1
  [yaw] -> Rate Command Direction Hold (RCDH)/3(psi0)
  Rate Command Direction Hold (RCDH)/1(psi) -> Mux/2
  [dir] -> Scaling/1
  Rate Command Height Hold (RCHH)/1(h) -> Altitude/1
  [h] -> Rate Command Height Hold (RCHH)/3(h0)
  [eta] -> Rate Command Height Hold (RCHH)/2(eta)
  [AltitudeRateComm] -> Rate Command Height Hold (RCHH)/1(h dot)
  h/1 -> [h]
  Data Type Conversion/1 -> Mux3/6
  [vert] -> Mux3/5
  [TRC] -> Data Type Conversion/1
  [fwd] -> Mux3/4
  [dir] -> Mux3/3
  [long] -> Mux3/2
  [lat] -> Mux3/1
  Mux3/1 -> To Workspace/1  "LatLonDirFwdVelVertVTRC"
  Subsystem/1(Velocity) -> Velocity/1
  [fwd] -> Subsystem/1(Fwd prop)
  beta/1 -> [beta]
  Turn Coordination (TC)/1(r_comm) -> r_comm/1
  [beta] -> Turn Coordination (TC)/2(Beta)
  [Vel] -> Turn Coordination (TC)/5(V)
  Constant2/1 -> Turn Coordination (TC)/3(g)
  Scaling2/1 -> Turn Coordination (TC)/1(Beta_comm)
  [euler] -> Turn Coordination (TC)/4(euler)
  kts2fts1/1 -> [xy_dot_comm]
  fts2kts/1 -> GreaterThan1/1
  [TRC_Flag] -> Translational Rate Command (TRC)/5(TRC Switch)
  AND1/1 -> [TRC_Flag], Sum9/1
  [Vel] -> fts2kts/1
  Constant3/1 -> GreaterThan1/2
  [TRC] -> AND1/1
  GreaterThan1/1 -> AND1/2
  Translational Rate Command (TRC)/1(RollPitchReq) -> [RP_TRC]
  Vel/1 -> [Vel]
  TRC/1 -> [TRC]
  [Vel_bEh] -> Translational Rate Command (TRC)/3(Vel_bEh)
  Vel_bEh/1 -> [Vel_bEh]
  Mux1/1 -> Scaling4/1
  AxisCorrection/1 -> Mux1/1
  Scaling4/1 -> kts2fts1/1
  [long] -> AxisCorrection/1
  [AltitudeRateComm] -> Translational Rate Command (TRC)/2(z_dot_req)
  [xy_dot_comm] -> Translational Rate Command (TRC)/1(xy_dot_comm)
  [lat] -> Mux1/2
  [long] -> Scaling5/1
  Lateral/1 -> [lat]
  Longitudinal/1 -> [long]
  [dir] -> Scaling2/1
  Mux/1 -> RollPitchYaw/1
  Directional/1 -> [dir]
  euler/1 -> [euler]
  eta/1 -> [eta]
  Fwd prop/1 -> [fwd]
  [yaw] -> Translational Rate Command (TRC)/4(yaw)

== system VehicleSimulationRef/ADCL Vehicle Control/Reference model ==
  rpy_comm : Inport
  h_comm : Inport  Port=2
  v_comm : Inport  Port=3
  r_comm : Inport  Port=4
  (2*damp*omega) : Gain  Gain=2*damp.*omega
  Constant : Constant  Value=0
  Constant1 : Constant  Value=0
  Integrator3 : Integrator  InitialCondition=[SimIn.IC.phi; SimIn.IC.theta; wrapToPi(SimIn.IC.psi); SimIn.EOM.Pos_bii(3); SimIn.IC.Vtot]  UpperSaturationLimit=deg2rad([28.5;15;inf;inf;inf])  LowerSaturationLimit=-deg2rad([28.5;15;inf;inf;inf])
  Integrator4 : Integrator  InitialCondition=[SimIn.IC.phidot; SimIn.IC.thetadot; SimIn.IC.psidot; SimIn.EOM.Vel_bIi(3); 0]  UpperSaturationLimit=deg2rad([5;5;inf;inf;inf])  LowerSaturationLimit=-deg2rad([5;5;inf;inf;inf])
  Mux : Mux  Inputs=3
  Mux1 : Mux  Inputs=2
  Mux2 : Mux  Inputs=2
  Mux3 : Mux  Inputs=2
  Subsystem : Subsystem
  Sum5 : Sum  Inputs=|+-
  Sum7 : Sum  Inputs=|+-
  omega/(2*damp) : Gain  Gain=omega./(2*damp)
  ref : Outport
  ref_dot : Outport  Port=2
  ref_ddot : Outport  Port=3
  wires:
  Subsystem/1(ref_out) -> ref/1
  Mux1/1 -> Subsystem/1(ref_in)
  rpy_comm/1 -> Mux/1
  h_comm/1 -> Mux/2
  Sum5/1 -> omega/(2*damp)/1
  Sum7/1 -> (2*damp*omega)/1
  omega/(2*damp)/1 -> Sum7/1
  (2*damp*omega)/1 -> Mux3/1, Integrator4/1
  Mux/1 -> Sum5/1
  Integrator3/1 -> Mux1/1, Sum5/2
  Integrator4/1 -> Mux2/1, Integrator3/1, Sum7/2
  v_comm/1 -> Mux/3, Subsystem/2(v_comm)
  r_comm/1 -> Mux1/2
  Mux2/1 -> ref_dot/1
  Mux3/1 -> ref_ddot/1
  Constant1/1 -> Mux3/2
  Constant/1 -> Mux2/2

== system VehicleSimulationRef/ADCL Vehicle Control/Variant Subsystem ==
  note: 1) Add Subsystem or Model blocks as valid variant choices.
      | 2) You cannot connect blocks at this level. At simulation, connectivity is automatically
      | determined, based on the active variant and port name matching.
  EOM : Inport
  eta : Inport  Port=2
  vtol_state : Inport  Port=3
  AutoFlight : Subsystem  VariantControl=SimIn.ctrlMode == CtrlModeEnum.Autonomous
  Local Pilot : Subsystem  VariantControl=SimIn.ctrlMode == CtrlModeEnum.LocalPilot
  Remote Pilot : Subsystem  VariantControl=SimIn.ctrlMode == CtrlModeEnum.RemotePilot
  fw_requested : Outport
  Lateral : Outport  Port=2
  Longitudinal : Outport  Port=3
  Directional : Outport  Port=4
  Vert prop : Outport  Port=5
  Fwd prop : Outport  Port=6
  TRC : Outport  Port=7
  RCAH : Outport  Port=8

== system VehicleSimulationRef/ADCL Vehicle Control/Mapping To Output/Eng Dynamics Compensation ==
  note: 1) Add Subsystem or Model blocks as valid variant choices.
      | 2) You cannot connect blocks at this level. At simulation, connectivity is automatically
      | determined, based on the active variant and port name matching.
  Eng_Des : Inport
  Default : Subsystem  VariantControl=SimIn.propType == 1
  First Order : Subsystem  VariantControl=SimIn.propType == 2 || SimIn.propType == 4
  Eng_Cmd : Outport

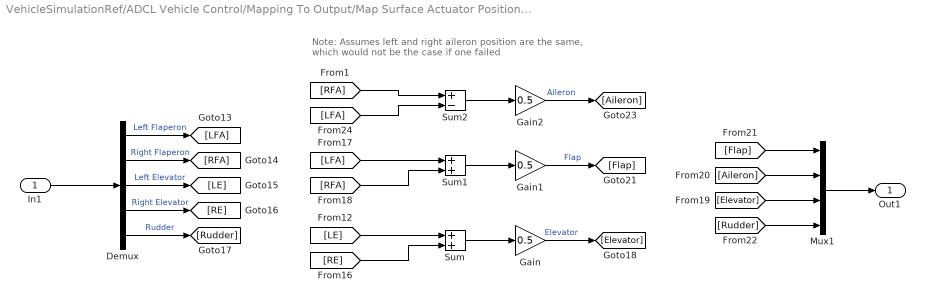
== system VehicleSimulationRef/ADCL Vehicle Control/Mapping To Output/Map Surface Actuator Position To Surface Inputs ==
  note: Note:  Assumes left and right aileron position are the same,
      |           which would not be the case if one failed
  In1 : Inport
  Demux : Demux  Outputs=SimIn.numSurfaces
  Gain : Gain  Gain=0.5
  Gain1 : Gain  Gain=0.5
  Gain2 : Gain  Gain=0.5
  Mux1 : Mux
  Sum : Sum
  Sum1 : Sum
  Sum2 : Sum  Inputs=+-
  Out1 : Outport
  wires:
  Gain2/1 -> [Aileron]  "Aileron"
  In1/1 -> Demux/1
  [LFA] -> Sum2/2
  Sum/1 -> Gain/1
  [RE] -> Sum/2
  Demux/3 -> [LE]  "Left Elevator"
  [LFA] -> Sum1/1
  Sum1/1 -> Gain1/1
  Sum2/1 -> Gain2/1
  Demux/4 -> [RE]  "Right Elevator"
  Gain/1 -> [Elevator]  "Elevator"
  [Rudder] -> Mux1/4
  Demux/5 -> [Rudder]  "Rudder"
  Demux/2 -> [RFA]  "Right Flaperon"
  [RFA] -> Sum1/2
  Mux1/1 -> Out1/1
  Demux/1 -> [LFA]  "Left Flaperon"
  [RFA] -> Sum2/1
  [LE] -> Sum/1
  [Elevator] -> Mux1/3
  Gain1/1 -> [Flap]  "Flap"
  [Aileron] -> Mux1/2
  [Flap] -> Mux1/1

== system VehicleSimulationRef/ADCL Vehicle Control/Mapping To Output/Surf Dynamics Compensation ==
  note: 1) Add Subsystem or Model blocks as valid variant choices.
      | 2) You cannot connect blocks at this level. At simulation, connectivity is automatically
      | determined, based on the active variant and port name matching.
  Surf_Des : Inport  PortDimensions=5
  Default : Subsystem  VariantControl=SimIn.actType == 1
  First Order : Subsystem  VariantControl=SimIn.actType == 2 || SimIn.actType == 4
  Surf_Cmd : Outport  PortDimensions=5

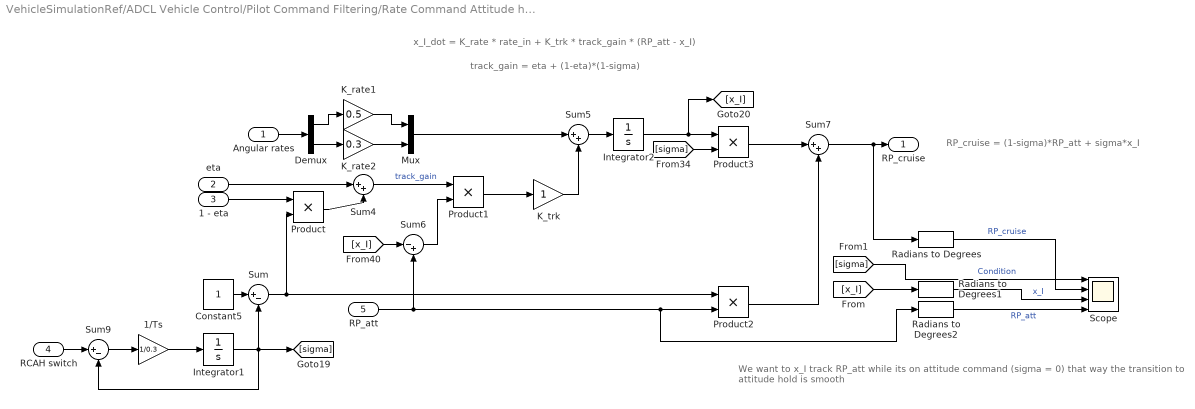
== system VehicleSimulationRef/ADCL Vehicle Control/Pilot Command Filtering/Rate Command Attitude hold (RCAH) ==
  note: RP_cruise = (1-sigma)*RP_att + sigma*x_I
  note: x_I_dot = K_rate * rate_in + K_trk * track_gain * (RP_att - x_I)
  note: track_gain = eta + (1-eta)*(1-sigma)
  note: We want to x_I track RP_att while its on attitude command (sigma = 0) that way the transition to attitude hold is smooth
  Angular rates : Inport
  eta : Inport  Port=2
  1 - eta : Inport  Port=3
  RCAH switch : Inport  Port=4
  RP_att : Inport  Port=5
  1/Ts : Gain  Gain=1/0.3
  Constant5 : Constant
  Demux : Demux  Outputs=2
  Integrator1 : Integrator
  Integrator2 : Integrator  LimitOutput=on  UpperSaturationLimit=[35; 30]*pi/180  LowerSaturationLimit=-[35; 30]*pi/180
  K_rate1 : Gain  Gain=0.5
  K_rate2 : Gain  Gain=0.3
  K_trk : Gain
  Mux : Mux  Inputs=2
  Product{,1..3} (4 alike) : Product
  Radians to Degrees : simulink_extras/Transformations/Radians to Degrees
  Radians to Degrees1 : simulink_extras/Transformations/Radians to Degrees
  Radians to Degrees2 : simulink_extras/Transformations/Radians to Degrees
  Scope : Scope  NumInputPorts=4
  Sum : Sum  Inputs=|+-
  Sum4 : Sum  Inputs=|++
  Sum5 : Sum  Inputs=|++
  Sum6 : Sum  Inputs=|-+
  Sum7 : Sum  Inputs=|++
  Sum9 : Sum  Inputs=|+-
  RP_cruise : Outport
  wires:
  K_rate2/1 -> Mux/2
  K_rate1/1 -> Mux/1
  Demux/2 -> K_rate2/1
  Demux/1 -> K_rate1/1
  Radians to Degrees/1 -> Scope/2  "RP_cruise"
  Radians to Degrees1/1 -> Scope/3  "x_I"
  Radians to Degrees2/1 -> Scope/4  "RP_att"
  [sigma] -> Scope/1  "Condition"
  [x_I] -> Radians to Degrees1/1
  Sum4/1 -> Product1/1  "track_gain"
  eta/1 -> Sum4/1
  Sum/1 -> Product/2, Product2/1
  1 - eta/1 -> Product/1
  K_trk/1 -> Sum5/2
  Product3/1 -> Sum7/1
  Product2/1 -> Sum7/2
  [sigma] -> Product3/2
  Integrator1/1 -> Sum9/2, [sigma], Sum/2
  Product/1 -> Sum4/2
  Mux/1 -> Sum5/1
  RP_att/1 -> Sum6/2, Product2/2, Radians to Degrees2/1
  Sum7/1 -> RP_cruise/1, Radians to Degrees/1
  Sum5/1 -> Integrator2/1
  Angular rates/1 -> Demux/1
  RCAH switch/1 -> Sum9/1
  Sum6/1 -> Product1/2
  Sum9/1 -> 1/Ts/1
  [x_I] -> Sum6/1
  Product1/1 -> K_trk/1
  Constant5/1 -> Sum/1
  1/Ts/1 -> Integrator1/1
  Integrator2/1 -> [x_I], Product3/1

== system VehicleSimulationRef/ADCL Vehicle Control/Pilot Command Filtering/Rate Command Direction Hold (RCDH) ==
  psi dot : Inport
  1 - eta : Inport  Port=2
  psi0 : Inport  Port=3
  Constant1 : Constant  Value=0
  Integrator1 : Integrator  ExternalReset=level  InitialConditionSource=external  UpperSaturationLimit=deg2rad(175)  LowerSaturationLimit=-deg2rad(175)  WrapState=on
  Switch : Switch  Criteria=u2 ~= 0  SaturateOnIntegerOverflow=off  InputSameDT=off
  psi : Outport
  wires:
  Constant1/1 -> Switch/1
  psi dot/1 -> Switch/3
  Switch/1 -> Integrator1/1
  Integrator1/1 -> psi/1
  psi0/1 -> Integrator1/3
  1 - eta/1 -> Integrator1/2, Switch/2

== system VehicleSimulationRef/ADCL Vehicle Control/Pilot Command Filtering/Rate Command Height Hold (RCHH) ==
  h dot : Inport
  eta : Inport  Port=2
  h0 : Inport  Port=3
  Integrator : Integrator  ExternalReset=rising  InitialConditionSource=external  InitialCondition=SimPar.EOM.Pos_bii(3)  LimitOutput=on  UpperSaturationLimit=0
  h : Outport
  wires:
  Integrator/1 -> h/1
  eta/1 -> Integrator/2
  h dot/1 -> Integrator/1
  h0/1 -> Integrator/3

== system VehicleSimulationRef/ADCL Vehicle Control/Pilot Command Filtering/Subsystem ==
  note: AutoFlight mode: Velocity dot req
      | Manual mode: Velocity
      | In AutoFlight mode we avoid the mapping
  note: (fwd_prop * (maxVel - minVel) + minVel ) * kts2fts * scale
  Fwd prop : Inport
  Constant : Constant  Commented=on  Value=100
  Constant1 : Constant  Commented=on  Value=SimIn.ctrlMode == CtrlModeEnum.Autonomous
  Product : Product
  Saturation1 : Saturate  UpperLimit=max(SimIn.CtrlTrim.trim_vel)  LowerLimit=SimIn.CtrlTrim.V_hover_exit
  Sum : Sum  Inputs=|++
  Sum1 : Sum  Inputs=|+-
  Switch : Switch  Commented=on  Criteria=u2 ~= 0  SaturateOnIntegerOverflow=off  InputSameDT=off
  VTOLScale : Gain  Gain=sqrt(SimPar.Scale)
  kts2fts : Gain  Gain=SimIn.Units.knot
  maxVel : Constant  Value=max(SimIn.CtrlTrim.trim_vel)
  minVel : Constant  Value=SimIn.CtrlTrim.V_hover_exit
  Velocity : Outport
  wires:
  Sum/1 -> Saturation1/1
  maxVel/1 -> Sum1/1
  Sum1/1 -> Product/2
  minVel/1 -> Sum/2, Sum1/2
  Product/1 -> Sum/1
  Constant1/1 -> Switch/2
  VTOLScale/1 -> Switch/3, Velocity/1
  kts2fts/1 -> VTOLScale/1
  Fwd prop/1 -> Product/1, Switch/1
  Saturation1/1 -> kts2fts/1

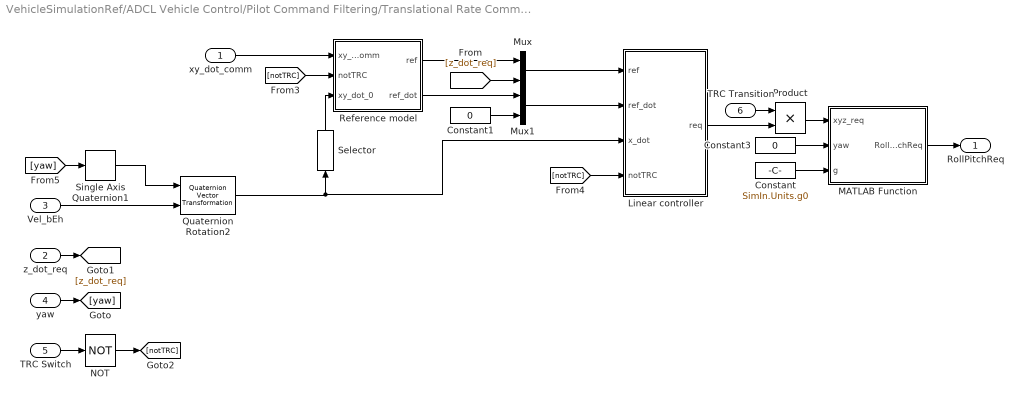
== system VehicleSimulationRef/ADCL Vehicle Control/Pilot Command Filtering/Translational Rate Command (TRC) ==
  xy_dot_comm : Inport
  z_dot_req : Inport  Port=2
  Vel_bEh : Inport  Port=3
  yaw : Inport  Port=4
  TRC Switch : Inport  Port=5
  TRC Transition : Inport  Port=6
  Constant : Constant  Value=SimIn.Units.g0
  Constant1 : Constant  Value=0
  Constant3 : Constant  Value=0
  Linear controller : Subsystem  mask{Kp=[0.5; 0.5; 0.5], Ki=[0.25^2; 0.25^2; 0], Ka=[1; 1; 0]}
      mask prompts: Kp "Rate gain"; Ki "Rate integral gain"; Ka "Acceleration gain"
      mask DialogControl DescTextVar Prompt: Linear controllers of the two TRC channels
  MATLAB Function : MATLAB Function  TreatAsAtomicUnit=on
  Mux : Mux  Inputs=2
  Mux1 : Mux  Inputs=2
  NOT : Logic  Operator=NOT  IconShape=distinctive  AllPortsSameDT=off  OutDataTypeStr=boolean
  Product : Product
  Quaternion Rotation2 : starslibAxisTransformations/Quaternion Vector Transformation  n=0
  Reference model : Subsystem  mask{Tv=3}
      mask prompts: Tv "Time constant"
      mask DialogControl DescTextVar Prompt: First order reference models for the two TRC channels
  Selector : Selector  InputPortWidth=3  IndexOptions=Index vector (dialog)  Indices=[1 2]  OutputSizes=1
  Single Axis Quaternion1 : starslibAxisTransformations/Single Axis Quaternion  RotAxis=z  n=0
  RollPitchReq : Outport
  wires:
  xy_dot_comm/1 -> Reference model/1(xy_dot_comm)
  Constant3/1 -> MATLAB Function/2(yaw)
  Quaternion Rotation2/1 -> Selector/1, Linear controller/3(x_dot)
  Vel_bEh/1 -> Quaternion Rotation2/2
  Single Axis Quaternion1/1 -> Quaternion Rotation2/1
  [yaw] -> Single Axis Quaternion1/1
  TRC Transition/1 -> Product/1
  Linear controller/1(req) -> Product/2
  Product/1 -> MATLAB Function/1(xyz_req)
  Selector/1 -> Reference model/3(xy_dot_0)
  MATLAB Function/1(RollPitchReq) -> RollPitchReq/1
  TRC Switch/1 -> NOT/1
  [notTRC] -> Linear controller/4(notTRC)
  [notTRC] -> Reference model/2(notTRC)
  NOT/1 -> [notTRC]
  [z_dot_req] -> Mux/2
  z_dot_req/1 -> [z_dot_req]
  yaw/1 -> [yaw]
  Constant1/1 -> Mux1/2
  Reference model/1(ref) -> Mux/1
  Mux1/1 -> Linear controller/2(ref_dot)
  Reference model/2(ref_dot) -> Mux1/1
  Mux/1 -> Linear controller/1(ref)
  Constant/1 -> MATLAB Function/3(g)

== system VehicleSimulationRef/ADCL Vehicle Control/Pilot Command Filtering/Turn Coordination (TC) ==
  Beta_comm : Inport
  Beta : Inport  Port=2
  g : Inport  Port=3
  euler : Inport  Port=4
  V : Inport  Port=5
  Constant : Constant  Value=0
  Demux : Demux  Outputs=3
  Divide : Product  Inputs=***/
  Gain : Gain  Gain=Kbeta
  IsNaN : RelationalOperator  Operator=isNaN  OutDataTypeStr=boolean  RndMeth=Simplest  InputSameDT=off
  IsNaN1 : RelationalOperator  Operator=isInf  OutDataTypeStr=boolean  RndMeth=Simplest  InputSameDT=off
  OR : Logic  Operator=OR  IconShape=distinctive  AllPortsSameDT=off  OutDataTypeStr=boolean
  Sin : Trigonometry
  Sin1 : Trigonometry  Operator=cos
  Sum : Sum  Inputs=|+-
  Sum1 : Sum  Inputs=|-+
  Switch : Switch  Criteria=u2 > Threshold  SaturateOnIntegerOverflow=off  InputSameDT=off
  Terminator : Terminator
  r_comm : Outport
  wires:
  OR/1 -> Switch/2
  IsNaN1/1 -> OR/2
  Beta_comm/1 -> Sum/1
  Beta/1 -> Sum/2
  Sum/1 -> Gain/1
  euler/1 -> Demux/1
  Demux/1 -> Sin/1
  Demux/2 -> Sin1/1
  g/1 -> Divide/1
  Sin/1 -> Divide/2
  Sin1/1 -> Divide/3
  V/1 -> Divide/4
  Divide/1 -> Sum1/2
  Demux/3 -> Terminator/1
  Gain/1 -> Sum1/1
  Switch/1 -> r_comm/1
  IsNaN/1 -> OR/1
  Sum1/1 -> IsNaN/1, IsNaN1/1, Switch/3
  Constant/1 -> Switch/1

== system VehicleSimulationRef/ADCL Vehicle Control/Reference model/Subsystem ==
  note: AutoFlight mode: Velocity dot req
      | Manual mode: Velocity
      | In AutoFlight mode we avoid the reference
      | model and use the raw signal directly
  ref_in : Inport
  v_comm : Inport  Port=2
  Constant1 : Constant  Value=SimIn.ctrlMode == CtrlModeEnum.Autonomous
  Mux : Mux  Inputs=3
  Selector : Selector  InputPortWidth=6  IndexOptions=Index vector (dialog)  Indices=1:4  OutputSizes=1
  Selector1 : Selector  InputPortWidth=6  IndexOptions=Index vector (dialog)  Indices=6  OutputSizes=1
  Switch : Switch  Criteria=u2 ~= 0  SaturateOnIntegerOverflow=off  InputSameDT=off
  ref_out : Outport
  wires:
  v_comm/1 -> Mux/2
  Mux/1 -> Switch/1
  Constant1/1 -> Switch/2
  Selector1/1 -> Mux/3
  Selector/1 -> Mux/1
  ref_in/1 -> Switch/3, Selector1/1, Selector/1
  Switch/1 -> ref_out/1

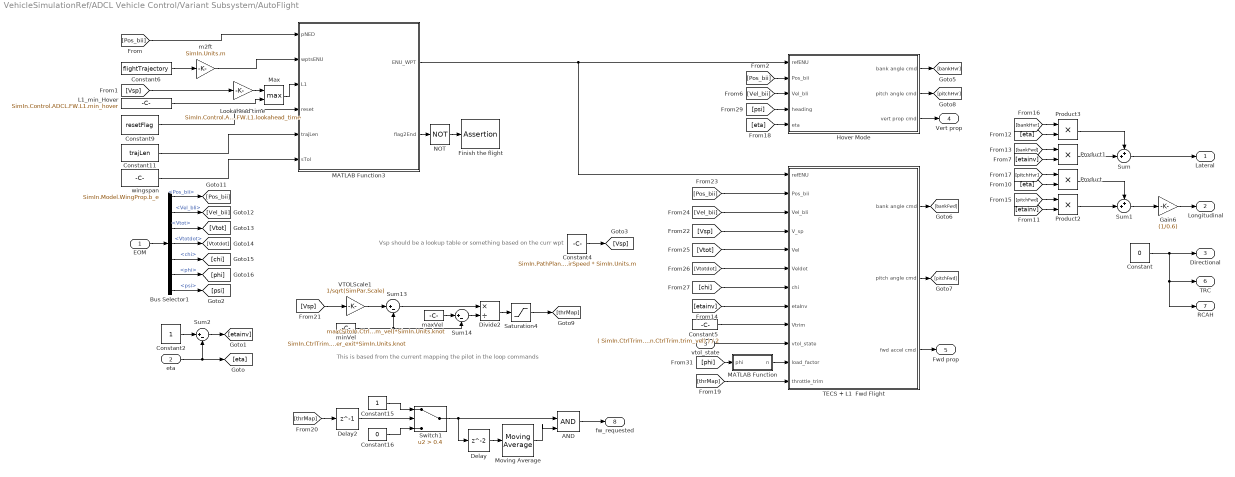
== system VehicleSimulationRef/ADCL Vehicle Control/Variant Subsystem/AutoFlight ==
  note: This is based from the current mapping the pilot in the loop commands
  note: Vsp should be a lookup table or something based on the curr wpt
  EOM : Inport
  eta : Inport  Port=2
  vtol_state : Inport  Port=3
  AND : Logic  IconShape=distinctive  AllPortsSameDT=off  OutDataTypeStr=boolean
  Bus Selector1 : BusSelector  OutputSignals=InertialData.Pos_bii,InertialData.Vel_bIi,AirRelativeData.Vtot,AirRelativeData.Vtotdot,WorldRelativeData.chi,WorldRelativeData.Euler.phi,WorldRelativeData.Euler.psi
  Constant : Constant  Value=0
  Constant11 : Constant  Value=trajLen
  Constant15 : Constant
  Constant16 : Constant  Value=0
  Constant2 : Constant
  Constant4 : Constant  Value=SimIn.PathPlan.AirSpeed * SimIn.Units.m
  Constant5 : Constant  Value=( SimIn.CtrlTrim.V_cruise_enter + max(SimIn.CtrlTrim.trim_vel) ) / 2
  Constant6 : Constant  Value=flightTrajectory
  Constant9 : Constant  Value=resetFlag
  Delay : Delay  InputProcessing=Columns as channels (frame based)  SampleTime=SimIn.Environment.Turbulence.dT
  Delay2 : Delay  DelayLength=1
  Divide2 : Product  Inputs=*/
  Finish the flight : Assertion
  Gain6 : Gain  Gain=(1/0.6)
  Hover Mode : Subsystem
  L1_min_Hover : Constant  Value=SimIn.Control.ADCL.FW.L1.min_hover
  Lookahead time : Gain  Gain=SimIn.Control.ADCL.FW.L1.lookahead_time
  MATLAB Function : MATLAB Function  TreatAsAtomicUnit=on
  MATLAB Function3 : MATLAB Function  TreatAsAtomicUnit=on
  Max : MinMax  Function=max  Inputs=2
  Moving Average : dspstat3/Moving Average  Method=Sliding window  ForgettingFactorPort=off  SpecifyWindowLength=on  WindowLength=50  OverlapLength=49  AllowArbitraryInputLength=off  ForgettingFactor=0.9  SimulateUsing=Interpreted execution
  NOT : Logic  Operator=NOT  IconShape=distinctive  AllPortsSameDT=off  OutDataTypeStr=boolean
  Product{,1..3} (4 alike) : Product
  Saturation4 : Saturate  UpperLimit=SimIn.Control.ADCL.FW.TECS.throttle_max  LowerLimit=SimIn.Control.ADCL.FW.TECS.throttle_min
  Sum : Sum  Inputs=++|
  Sum1 : Sum  Inputs=++|
  Sum13 : Sum  Inputs=|+-
  Sum14 : Sum  Inputs=|+-
  Sum2 : Sum  Inputs=|+-
  Switch1 : Switch  Criteria=u2 > Threshold  Threshold=0.4  SaturateOnIntegerOverflow=off  InputSameDT=off
  TECS + L1  Fwd Flight : Subsystem
  VTOLScale1 : Gain  Gain=1/sqrt(SimPar.Scale)
  m2ft : Gain  Gain=SimIn.Units.m
  maxVel : Constant  Value=max(SimIn.CtrlTrim.trim_vel)*SimIn.Units.knot
  minVel : Constant  Value=SimIn.CtrlTrim.V_hover_exit*SimIn.Units.knot
  wingspan : Constant  Value=SimIn.Model.WingProp.b_e
  Lateral : Outport
  Longitudinal : Outport  Port=2
  Directional : Outport  Port=3
  Vert prop : Outport  Port=4
  Fwd prop : Outport  Port=5
  TRC : Outport  Port=6
  RCAH : Outport  Port=7
  fw_requested : Outport  Port=8
  wires:
  [Pos_bii] -> Hover Mode/2(Pos_bii)
  Lookahead time/1 -> Max/1
  [Vsp] -> Lookahead time/1
  Constant11/1 -> MATLAB Function3/5(trajLen)
  Constant9/1 -> MATLAB Function3/4(reset)
  L1_min_Hover/1 -> Max/2
  Max/1 -> MATLAB Function3/3(L1)
  MATLAB Function3/2(flag2End) -> NOT/1
  NOT/1 -> Finish the flight/1
  MATLAB Function3/1(ENU_WPT) -> Hover Mode/1(refENU), TECS + L1  Fwd Flight/1(refENU)
  [Pos_bii] -> MATLAB Function3/1(pNED)
  Constant4/1 -> [Vsp]
  Bus Selector1/7 -> [psi]  "<psi>"
  TECS + L1  Fwd Flight/3(fwd accel cmd) -> Fwd prop/1
  [phi] -> MATLAB Function/1(phi)
  Bus Selector1/6 -> [phi]  "<phi>"
  [psi] -> Hover Mode/4(heading)
  [Vel_bii] -> Hover Mode/3(Vel_bIi)
  [Vtotdot] -> TECS + L1  Fwd Flight/6(Veldot)
  [Vtot] -> TECS + L1  Fwd Flight/5(Vel)
  [Vel_bii] -> TECS + L1  Fwd Flight/3(Vel_bIi)
  [chi] -> TECS + L1  Fwd Flight/7(chi)
  [Pos_bii] -> TECS + L1  Fwd Flight/2(Pos_bii)
  Bus Selector1/1 -> [Pos_bii]  "<Pos_bii>"
  Bus Selector1/2 -> [Vel_bii]  "<Vel_bIi>"
  Bus Selector1/3 -> [Vtot]  "<Vtot>"
  Bus Selector1/4 -> [Vtotdot]  "<Vtotdot>"
  Bus Selector1/5 -> [chi]  "<chi>"
  [Vsp] -> TECS + L1  Fwd Flight/4(V_sp)
  [thrMap] -> Delay2/1
  [thrMap] -> TECS + L1  Fwd Flight/12(throttle_trim)
  Saturation4/1 -> [thrMap]
  minVel/1 -> Sum13/2, Sum14/2
  maxVel/1 -> Sum14/1
  [Vsp] -> VTOLScale1/1
  VTOLScale1/1 -> Sum13/1
  Sum13/1 -> Divide2/1
  Divide2/1 -> Saturation4/1
  Sum14/1 -> Divide2/2
  vtol_state/1 -> TECS + L1  Fwd Flight/10(vtol_state)
  AND/1 -> fw_requested/1
  Moving Average/1 -> AND/2
  Delay/1 -> Moving Average/1
  Delay2/1 -> Switch1/2
  Switch1/1 -> AND/1, Delay/1
  Constant16/1 -> Switch1/3
  Constant15/1 -> Switch1/1
  Gain6/1 -> Longitudinal/1
  MATLAB Function/1(n) -> TECS + L1  Fwd Flight/11(load_factor)
  Constant5/1 -> TECS + L1  Fwd Flight/9(Vtrim)
  [eta] -> Hover Mode/5(eta)
  [pitchHvr] -> Product/1
  [bankHvr] -> Product3/1
  Hover Mode/2(pitch angle cmd) -> [pitchHvr]
  Hover Mode/1(bank angle cmd) -> [bankHvr]
  [pitchFwd] -> Product2/1
  [bankFwd] -> Product1/1
  TECS + L1  Fwd Flight/2(pitch angle cmd) -> [pitchFwd]
  TECS + L1  Fwd Flight/1(bank angle cmd) -> [bankFwd]
  [etainv] -> TECS + L1  Fwd Flight/8(etaInv)
  Sum1/1 -> Gain6/1
  Sum/1 -> Lateral/1
  m2ft/1 -> MATLAB Function3/2(wptsENU)
  Constant2/1 -> Sum2/1
  Sum2/1 -> [etainv]
  Product2/1 -> Sum1/2
  Product1/1 -> Sum/2
  Product/1 -> Sum1/1
  Product3/1 -> Sum/1
  [eta] -> Product3/2
  [etainv] -> Product2/2
  [etainv] -> Product1/2
  [eta] -> Product/2
  eta/1 -> [eta], Sum2/2
  Constant6/1 -> m2ft/1
  Hover Mode/3(vert prop cmd) -> Vert prop/1
  Constant/1 -> Directional/1, TRC/1, RCAH/1
  EOM/1 -> Bus Selector1/1
  wingspan/1 -> MATLAB Function3/6(sTol)
